simulink model "finalmodel"  (R2015a)
settings: Solver=ode3  StartTime=0.0  StopTime=5  FixedStep=0.00001  RelTol=1e-3
values from neighbouring files (symbols this model uses):
  g = 9.81    [controlmodeltestspoleplacment.m]    (also in controlwithintegratorsLQR.m; controlwithoutencoderonlyMPUgains.m)
  K = place(A,B,[p1, p2, p3,p4])    [controlmodeltestspoleplacment.m]    (also in controlwithintegratorsLQR.m = lqr(A,B,Q,RR); controlwithoutencoderonlyMPUgains.m = lqr(A,B,Q,RR))
  L = 0.080    (= 0.08)    [controlmodeltestspoleplacment.m]    (also in controlwithintegratorsLQR.m = 0.11; controlwithoutencoderonlyMPUgains.m = 0.068)
  m = (y(:,2)./r)-y(:,4)    [controlwithintegratorsLQR.m]
  Nbar = K(1)    [controlmodeltestspoleplacment.m]    (also in controlwithintegratorsLQR.m; controlwithoutencoderonlyMPUgains.m = K(3))
  R = 5.6/48    (= 0.116666666667)    [controlmodeltestspoleplacment.m]    (also in controlwithintegratorsLQR.m; controlwithoutencoderonlyMPUgains.m)
undefined symbols (not defined in the file or in its folder): fm_l, fm_r, J_eps, J_phi, Jw_l, Jw_r, Kb_l, Kb_r, Kt_l, Kt_r, M, n, R_a, W
libraries: simulink x2
settings Model: Creator=omaRhagrass  LastModifiedBy=omaRhagrass
settings SolverCC: AlgebraicLoopSolver=LineSearch  PositivePriorityOrder=on  AutoInsertRateTranBlk=on
settings DataIOCC: LimitDataPoints=off
settings OptimizationCC: InlineParams=on  BufferReuse=off
settings DebuggingCC: InitInArrayFormatMsg=none

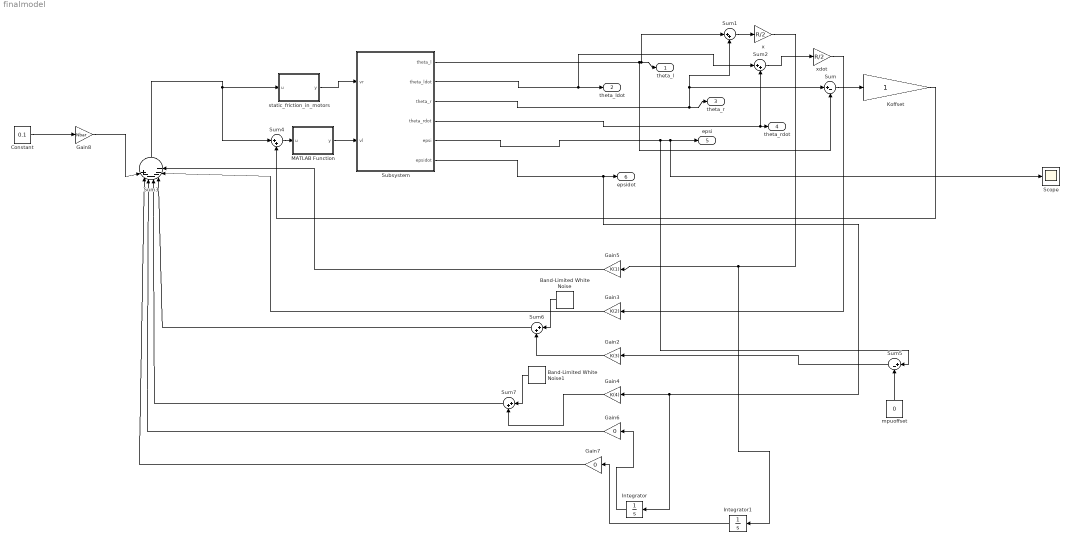
== system finalmodel ==
  Band-Limited White Noise : simulink/Sources/Band-Limited White Noise  Cov=[0.1]  Ts=0.1  seed=[23341]
  Band-Limited White Noise1 : simulink/Sources/Band-Limited White Noise  Cov=[0.1]  Ts=0.1  seed=[23341]
  Constant : Constant  Value=0.1
  Gain2 : Gain  Gain=K(3)
  Gain3 : Gain  Gain=K(2)
  Gain4 : Gain  Gain=K(4)
  Gain5 : Gain  Gain=K(1)
  Gain6 : Gain  Gain=0
  Gain7 : Gain  Gain=0
  Gain8 : Gain  Gain=Nbar
  Integrator : Integrator
  Integrator1 : Integrator
  Koffset : Gain
  MATLAB Function : MATLAB Function  TreatAsAtomicUnit=on
  Scope : Scope
  Subsystem : Subsystem
  Sum : Sum  Inputs=|+-
  Sum{1..2,4,6..7} (5 alike) : Sum  Inputs=|++
  Sum3 : Sum  Inputs=|+------
  Sum5 : Sum  Inputs=|+-
  "mpuoffset " : Constant  Value=0
  static_friction_in_motors : MATLAB Function  TreatAsAtomicUnit=on
  x : Gain  Gain=R/2
  xdot : Gain  Gain=R/2
  "theta_l " : Outport
  "theta_ldot " : Outport  Port=2
  "theta_r " : Outport  Port=3
  "theta_rdot " : Outport  Port=4
  "epsi " : Outport  Port=5
  "epsidot " : Outport  Port=6
  wires:
  Sum3/1 -> Sum4/1, static_friction_in_motors/1(u)
  Subsystem/1("theta_l ") -> Sum/2, Sum1/1, "theta_l "/1
  Subsystem/3("theta_r ") -> Sum1/2, Sum/1, "theta_r "/1
  Subsystem/4("theta_rdot ") -> Sum2/2, "theta_rdot "/1
  Subsystem/5("epsi ") -> Sum5/1, Scope/1, "epsi "/1
  Subsystem/6("epsidot ") -> Integrator/1, Gain4/1, "epsidot "/1
  Sum/1 -> Koffset/1
  Sum1/1 -> x/1
  Subsystem/2("theta_ldot ") -> Sum2/1, "theta_ldot "/1
  Sum2/1 -> xdot/1
  xdot/1 -> Gain3/1
  Integrator/1 -> Gain6/1
  x/1 -> Integrator1/1, Gain5/1
  Integrator1/1 -> Gain7/1
  Gain7/1 -> Sum3/2
  Gain6/1 -> Sum3/3
  Gain3/1 -> Sum3/6
  Gain5/1 -> Sum3/7
  Constant/1 -> Gain8/1
  Gain8/1 -> Sum3/1
  Koffset/1 -> Sum4/2
  Sum4/1 -> MATLAB Function/1(u)
  MATLAB Function/1(y) -> Subsystem/2("vl ")
  static_friction_in_motors/1(y) -> Subsystem/1(vr)
  Sum5/1 -> Gain2/1
  "mpuoffset "/1 -> Sum5/2
  Band-Limited White Noise/1 -> Sum6/1
  Gain2/1 -> Sum6/2
  Sum6/1 -> Sum3/5
  Band-Limited White Noise1/1 -> Sum7/1
  Sum7/1 -> Sum3/4
  Gain4/1 -> Sum7/2

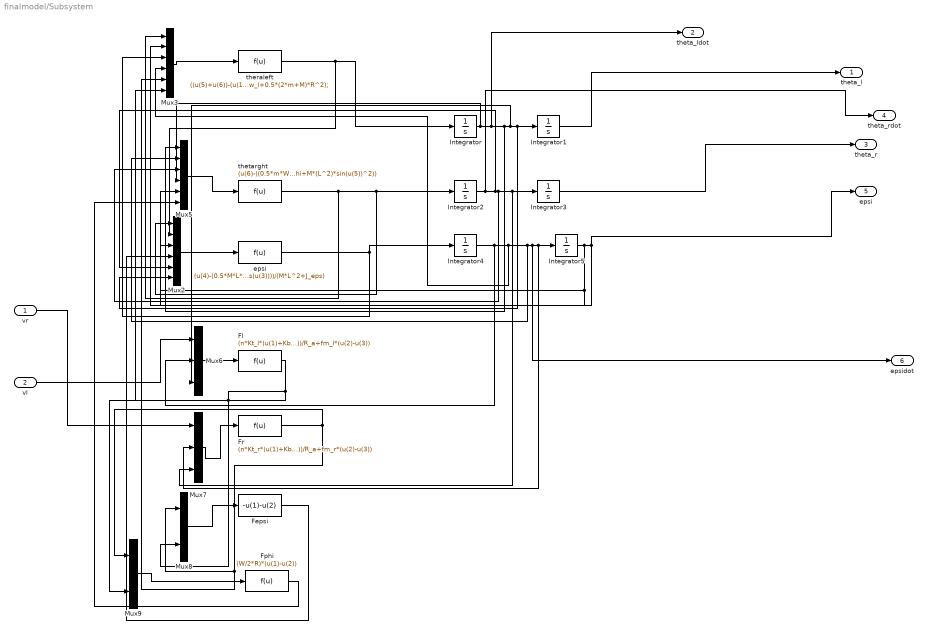
== system finalmodel/Subsystem ==
  vr : Inport
  "vl " : Inport  Port=2
  Fepsi : Fcn  Expr=-u(1)-u(2)
  Fl : Fcn  Expr=(n*Kt_l*(u(1)+Kb_l*(u(2)-u(3))*n))/R_a+fm_l*(u(2)-u(3))
  "Fphi " : Fcn  Expr=(W/2*R)*(u(1)-u(2))
  "Fr " : Fcn  Expr=(n*Kt_r*(u(1)+Kb_r*(u(2)-u(3))*n))/R_a+fm_r*(u(2)-u(3))
  Integrator{,1..5} (6 alike) : Integrator
  Mux2 : Mux  Inputs=6
  Mux3 : Mux  Inputs=6
  Mux5 : Mux  Inputs=6
  Mux6 : Mux  Inputs=3
  Mux7 : Mux  Inputs=3
  Mux8 : Mux  Inputs=2
  Mux9 : Mux  Inputs=2
  epsi : Fcn  Expr=(u(4)-(0.5*M*L*R*cos(u(3))*(u(1)+u(2))-M*g*L*sin(u(3))-M*(L^2)*((R/W)*(u(5)-u(6)))^2*sin(u(3))*cos(u(3))))/(M*L^2+J_eps)
  "theraleft " : Fcn  Expr=((u(5)+u(6))-(u(1)*0.5*(2*m+M)*(R^2)+Jw_r*u(1)+(M*L*R*cos(u(2)))*u(3)-M*L*R*u(4)^2*sin(u(2))))/(Jw_l+0.5*(2*m+M)*R^2);
  thetarght : Fcn  Expr=(u(6)-((0.5*m*W^2+J_phi+M*(L^2)*sin(u(5))^2)*(R/W)*-u(1)-(W/2*R)*Jw_l*u(1)+2*M*L^2*u(2)*(R/W)*(u(3)-u(4))*sin(u(5))*cos(u(5))))/((W/(2*R))*Jw_r+(R/W)*(0.5*m*W^2+J_phi+M*(L^2)*sin(u(5))^2))
  "theta_l " : Outport
  "theta_ldot " : Outport  Port=2
  "theta_r " : Outport  Port=3
  "theta_rdot " : Outport  Port=4
  "epsi " : Outport  Port=5
  "epsidot " : Outport  Port=6
  wires:
  Integrator1/1 -> "theta_l "/1
  "Fphi "/1 -> Mux5/6
  "theraleft "/1 -> Mux2/2, Integrator/1
  Integrator4/1 -> Mux6/2, Mux5/2, "epsidot "/1, Mux7/2, Integrator5/1, Mux3/4
  "vl "/1 -> Mux6/1
  Integrator5/1 -> Mux5/5, Mux2/3, "epsi "/1, Mux3/2
  Integrator/1 -> Mux5/4, "theta_ldot "/1, Mux5/1, Mux2/6, Integrator1/1, Mux6/3
  Integrator2/1 -> "theta_rdot "/1, Mux2/5, Mux5/3, Integrator3/1, Mux7/3
  Mux7/1 -> "Fr "/1
  Mux9/1 -> "Fphi "/1
  Integrator3/1 -> "theta_r "/1
  Mux8/1 -> Fepsi/1
  Mux3/1 -> "theraleft "/1
  epsi/1 -> Mux3/3, Integrator4/1
  Mux6/1 -> Fl/1
  Mux2/1 -> epsi/1
  thetarght/1 -> Mux3/1, Mux2/1, Integrator2/1
  Fl/1 -> Mux9/2, Mux3/6, Mux8/2
  "Fr "/1 -> Mux3/5, Mux8/1, Mux9/1
  Fepsi/1 -> Mux2/4
  vr/1 -> Mux7/1
  Mux5/1 -> thetarght/1

== matlab function finalmodel/static_friction_in_motors ==
  data: u input; y output
function y = fcn(u)
if(abs(u)<1)
y=0;
else
    y=u;
end
end

== matlab function finalmodel/MATLAB Function ==
  data: u input; y output
function y = fcn(u)
if(abs(u)<1)
y=0;
else
    y=u;
end
end
